simulink model "Murray_Mexp"  (Simulink 7.5)
settings: Solver=ode45  StartTime=0.0  StopTime=10.0  RelTol=1e-3
values from neighbouring files (symbols this model uses):
  apSampleTime = 0.01    [demoz2SlugsV5.m]
undefined symbols (not defined in the file or in its folder): apSampleT
libraries: dspmtrx3 x1
settings Model: Creator=Robert  LastModifiedBy=Robert

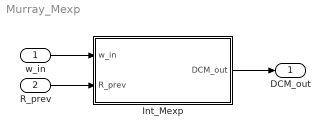
== system Murray_Mexp ==
  w_in : Inport  OutDataType=fixdt(1, 16)  OutScaling=2^0
  R_prev : Inport  Port=2  OutDataType=fixdt(1, 16)  OutScaling=2^0
  Int_Mexp : Subsystem
  DCM_out : Outport  OutDataType=fixdt(1, 16)  OutScaling=2^0
  wires:
  w_in/1 -> Int_Mexp/1(w_in)
  Int_Mexp/1(DCM_out) -> DCM_out/1
  R_prev/1 -> Int_Mexp/2(R_prev)

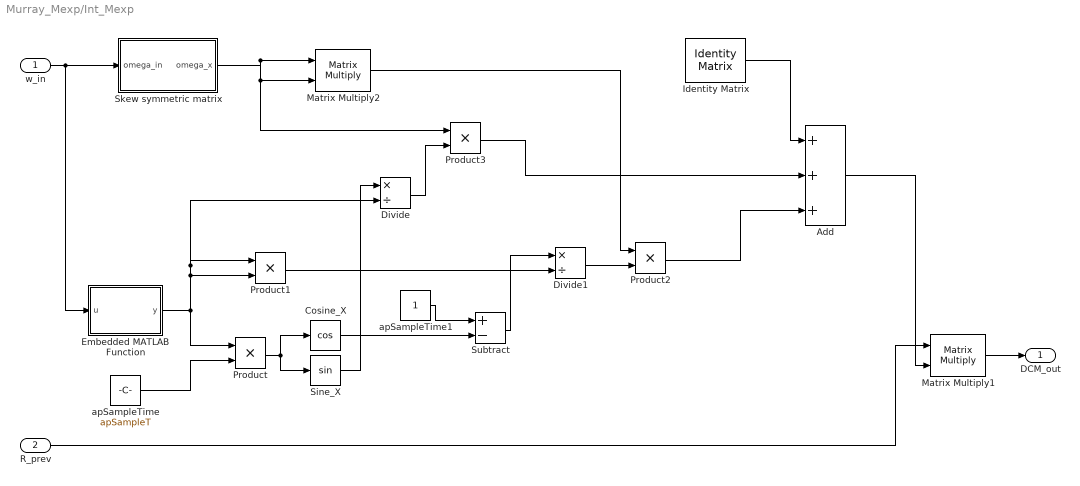
== system Murray_Mexp/Int_Mexp ==
  w_in : Inport  OutDataType=fixdt(1, 16)  OutScaling=2^0
  R_prev : Inport  Port=2  OutDataType=fixdt(1, 16)  OutScaling=2^0
  Add : Sum  Inputs=+++  OutDataTypeMode=single  OutDataType=fixdt(1, 16)  OutScaling=2^-10  OutDataTypeStr=single  SampleTime=apSampleTime
  Cosine_X : Trigonometry  Operator=cos
  Divide : Product  Inputs=*/  OutDataType=fixdt(1, 16)  OutScaling=2^-10
  Divide1 : Product  Inputs=*/  OutDataType=fixdt(1, 16)  OutScaling=2^-10
  Embedded MATLAB Function : Stateflow chart  TreatAsAtomicUnit=on
  Identity Matrix : dspmtrx3/Identity Matrix  Inherit=off  N=3  Ts=1  dataType=single  isSigned=on  wordLen=16  udDataType=sfix(16)  fracBitsMode=Best precision  numFracBits=15
  Matrix Multiply1 : Product  Multiplication=Matrix(*)  OutDataType=sfix(16)  OutScaling=2^0
  Matrix Multiply2 : Product  Multiplication=Matrix(*)  OutDataType=sfix(16)  OutScaling=2^0
  Product{,1..3} (4 alike) : Product  OutDataType=fixdt(1, 16)  OutScaling=2^0  RndMeth=Zero
  Sine_X : Trigonometry
  Skew symmetric matrix : Subsystem
  Subtract : Sum  Inputs=+-  OutDataType=fixdt(1, 16)  OutScaling=2^-10
  apSampleTime : Constant  Value=apSampleT  OutDataTypeMode=single  OutDataType=fixdt(1, 16)  OutScaling=2^0  OutDataTypeStr=single
  apSampleTime1 : Constant  OutDataTypeMode=single  OutDataType=fixdt(1, 16)  OutScaling=2^0  OutDataTypeStr=single
  DCM_out : Outport  OutDataType=fixdt(1, 16)  OutScaling=2^0
  wires:
  w_in/1 -> Embedded MATLAB Function/1(u), Skew symmetric matrix/1(omega_in)
  Identity Matrix/1 -> Add/1
  Embedded MATLAB Function/1(y) -> Product/1, Product1/2, Product1/1, Divide/2
  apSampleTime/1 -> Product/2
  Product/1 -> Cosine_X/1, Sine_X/1
  Skew symmetric matrix/1(omega_x) -> Matrix Multiply2/1, Matrix Multiply2/2, Product3/1
  apSampleTime1/1 -> Subtract/1
  Cosine_X/1 -> Subtract/2
  Subtract/1 -> Divide1/1
  Product1/1 -> Divide1/2
  Divide1/1 -> Product2/2
  Matrix Multiply2/1 -> Product2/1
  Product2/1 -> Add/3
  Sine_X/1 -> Divide/1
  Divide/1 -> Product3/2
  Product3/1 -> Add/2
  R_prev/1 -> Matrix Multiply1/1
  Add/1 -> Matrix Multiply1/2
  Matrix Multiply1/1 -> DCM_out/1

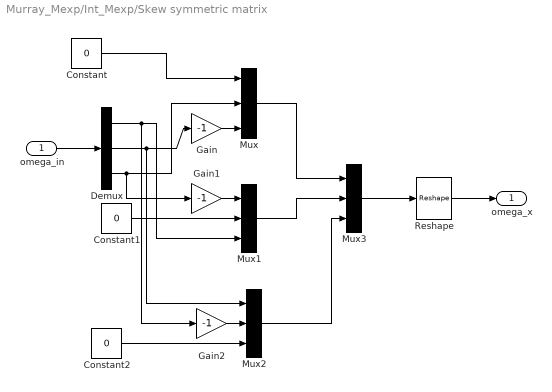
== system Murray_Mexp/Int_Mexp/Skew symmetric matrix ==
  omega_in : Inport  OutDataType=fixdt(1, 16)  OutScaling=2^0
  Constant : Constant  Value=0  OutDataType=fixdt(1, 16)  OutScaling=2^0
  Constant1 : Constant  Value=0  OutDataType=fixdt(1, 16)  OutScaling=2^0
  Constant2 : Constant  Value=0  OutDataType=fixdt(1, 16)  OutScaling=2^0
  Demux : Demux  Outputs=3
  Gain : Gain  Gain=-1  ParameterDataType=fixdt(1, 16)  ParameterScaling=2^0  OutDataType=fixdt(1, 16)  OutScaling=2^0
  Gain1 : Gain  Gain=-1  ParameterDataType=fixdt(1, 16)  ParameterScaling=2^0  OutDataType=fixdt(1, 16)  OutScaling=2^0
  Gain2 : Gain  Gain=-1  ParameterDataType=fixdt(1, 16)  ParameterScaling=2^0  OutDataType=fixdt(1, 16)  OutScaling=2^0
  Mux{,1..3} (4 alike) : Mux  Inputs=3
  Reshape : Reshape  OutputDimensionality=Customize  OutputDimensions=[3,3]
  omega_x : Outport  OutDataType=fixdt(1, 16)  OutScaling=2^0
  wires:
  omega_in/1 -> Demux/1
  Reshape/1 -> omega_x/1
  Constant/1 -> Mux/1
  Demux/3 -> Mux/2, Gain1/1
  Demux/2 -> Gain/1, Mux2/1
  Constant1/1 -> Mux1/2
  Demux/1 -> Mux1/3, Gain2/1
  Constant2/1 -> Mux2/3
  Mux/1 -> Mux3/1
  Mux1/1 -> Mux3/2
  Mux2/1 -> Mux3/3
  Mux3/1 -> Reshape/1
  Gain/1 -> Mux/3
  Gain1/1 -> Mux1/1
  Gain2/1 -> Mux2/2

== matlab function Int_Mexp/Embedded MATLAB Function ==
  data: u input double; y output double
function y = GetNorm(u)
%#eml
% Function returns the 2-norm of the input argument.

y = norm(u);
